simulink model "FreePortComm_RXTX"  (Simulink 7.4)
settings: Solver=FixedStepDiscrete  SolverMode=SingleTasking  StartTime=0.0  StopTime=inf  FixedStep=.02  RelTol=1e-3
settings Model: Creator=Admin  LastModifiedBy=fw  SimulationMode=external  ExtModeTrigDuration=500
settings ConfigSet: Description=rtmc9s12target_R2009b
settings DataIOCC: SignalLoggingName=sigsOut
settings OptimizationCC: BooleanDataType=off  InitFltsAndDblsToZero=on  OptimizeModelRefInitCode=on  LifeSpan=1
settings DebuggingCC: SaveWithParameterizedLinksMsg=none  SignalResolutionControl=TryResolveAllWithWarning  SolverPrmCheckMsg=none  MultiTaskDSMMsg=warning  MultiTaskCondExecSysMsg=none  StrictBusMsg=None
settings HardwareCC: ProdBitPerInt=16  ProdEndianess=BigEndian  ProdWordSize=16  ProdHWDeviceType=Motorola HC12
settings RTWCC: SystemTargetFile=mc9s12.tlc  GenerateMakefile=off  TemplateMakefile=mc9s12.tmf  ProcessScript=mc9s12_make_rtw_hook  IncludeERTFirstTime=on
settings CodeAppCC: IgnoreCustomStorageClasses=off
settings STFCustomTargetCC: TargetFcnLib=ansi_tfl_tmw.mat  ModelReferenceCompliant=off  IncludeMdlTerminateFcn=off  ERTCustomFileBanners=on  SupportNonInlinedSFcns=off  CPPClassGenCompliant=on  SystemTargetFile=mc9s12.tlc
settings ERTTargetCC: TargetFcnLib=ansi_tfl_tmw.mat  MultiwordLength=2048  ModelReferenceCompliant=off  ParMdlRefBuildCompliant=off  CompOptLevelCompliant=off  IncludeMdlTerminateFcn=off  CombineOutputUpdateFcns=off  ERTFirstTimeCompliant=off  SupportContinuousTime=on  ModelStepFunctionPrototypeControlCompliant=off  ExtModeMexFile=ext_serial_mc9s12_comm  ExtModeMexArgs=1,2,115200  InlinedParameterPlacement=NonHierarchical  ERTCustomFileTemplate=mc9s12_file_process.tlc  GRTInterface=on  ConvertIfToSwitch=off
settings CustomProperty: DataType=RTWOptions_EnumType_C__Users_fw__SVN_rtmc9s12-target_trunk_rtmc9s12_CW_R2009b_bin_mc9s12_1mc9s12_TargetBoard  Value=Dragon12Plus
settings EnumStrPairs: String=Dragon12

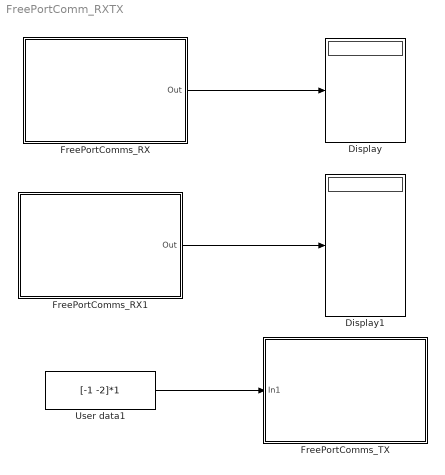
== system FreePortComm_RXTX ==
  Display : Display
  Display1 : Display
  FreePortComms_RX : Subsystem  Tag=mcTarget_freePortCommsRX  mask{sampletime=0.1, port=SCI0, baudrate=115200, channel=0, buf_size=5, data_type=UINT8, format=off, outformat=on}
      mask prompts: sampletime "Sample time"; port "Communication port"; channel "Channel number"; buf_size "Number of elements"; data_type "Data Type"; format "Block receives raw data"; outformat "Block output is double"
      mask init:
      | [buf_sizestr, portNamestr, baudratestr, channelstr, data_type_str, sampletime_str] = mbc_freeportrxd(sampletime, port, baudrate, channel, buf_size, data_type, format, outformat);
      mask Help: web('freePortComms_rxd.html');
      mask StyleString: edit,popup(SCI0|SCI1|COM1|COM2|COM3|COM4),popup(300|600|1200|2400|4800|9600|19200|38400|57600|115200),edit,edit,popup(SINGLE|INT8|UINT8|INT16|UINT16|INT32|UINT32|BOOLEAN),checkbox,checkbox
      mask Display: fprintf('Receive %s element(s)\nComm port: %s\nBaudrate: %s bps\nChannel: %s\nData type: %s\n Sample rate: %s', buf_sizestr, portNamestr, baudratestr, channelstr, data_type_str, sampletime_str)
  FreePortComms_RX1 : Subsystem  Tag=mcTarget_freePortCommsRX  mask{sampletime=0.1, port=SCI0, baudrate=115200, channel=1, buf_size=7, data_type=SINGLE, format=off, outformat=on}
      mask prompts: sampletime "Sample time"; port "Communication port"; channel "Channel number"; buf_size "Number of elements"; data_type "Data Type"; format "Block receives raw data"; outformat "Block output is double"
      mask init:
      | [buf_sizestr, portNamestr, baudratestr, channelstr, data_type_str, sampletime_str] = mbc_freeportrxd(sampletime, port, baudrate, channel, buf_size, data_type, format, outformat);
      mask Help: web('freePortComms_rxd.html');
      mask StyleString: edit,popup(SCI0|SCI1|COM1|COM2|COM3|COM4),popup(300|600|1200|2400|4800|9600|19200|38400|57600|115200),edit,edit,popup(SINGLE|INT8|UINT8|INT16|UINT16|INT32|UINT32|BOOLEAN),checkbox,checkbox
      mask Display: fprintf('Receive %s element(s)\nComm port: %s\nBaudrate: %s bps\nChannel: %s\nData type: %s\n Sample rate: %s', buf_sizestr, portNamestr, baudratestr, channelstr, data_type_str, sampletime_str)
  FreePortComms_TX : Subsystem  Tag=mcTarget_freePortCommsTX  mask{sampletime=0.1, port=SCI0, baudrate=115200, channel=3, buf_size=2, data_type=INT32, format=off}
      mask prompts: sampletime "Sample time"; port "Communication port"; channel "Channel number"; buf_size "Number of elements"; data_type "Data Type"; format "Block sends raw data"
      mask init:
      | [buf_sizestr, portNamestr, baudratestr, channelstr, data_type_str, sampletime_str] = mbc_freeporttxd(sampletime, port, baudrate, channel, buf_size, data_type, format);
      mask Help: web('freePortComms_txd.html');
      mask StyleString: edit,popup(SCI0|SCI1|COM1|COM2|COM3|COM4),popup(300|600|1200|2400|4800|9600|19200|38400|57600|115200),edit,edit,popup(SINGLE|INT8|UINT8|INT16|UINT16|INT32|UINT32|BOOLEAN),checkbox
      mask Display: fprintf('Transmit %s element(s)\nComm port: %s\nBaudrate: %s bps\nChannel: %s\nData type: %s\n Sample rate: %s', buf_sizestr, portNamestr, baudratestr, channelstr, data_type_str, sampletime_str)
  User data1 : Constant  Value=[-1 -2]*1  OutDataType=sfix(16)  OutScaling=2^0
  wires:
  FreePortComms_RX/1(Out) -> Display/1
  FreePortComms_RX1/1(Out) -> Display1/1
  User data1/1 -> FreePortComms_TX/1(In1)

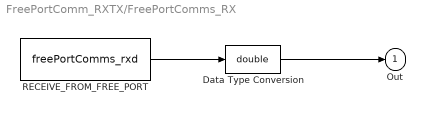
== system FreePortComm_RXTX/FreePortComms_RX ==
  Data Type Conversion : DataTypeConversion  OutDataTypeMode=double  OutDataType=sfix(16)  OutScaling=2^0  OutDataTypeStr=double  SaturateOnIntegerOverflow=on  RndMeth=Zero
  RECEIVE_FROM_FREE_PORT : S-Function  Tag=mcTarget_freePortCommsRX  FunctionName=freePortComms_rxd  Parameters=sampletime, channel, buf_size, data_type, port, baudrate, format  EnableBusSupport=off
  Out : Outport  OutDataType=sfix(16)  OutScaling=2^0
  wires:
  RECEIVE_FROM_FREE_PORT/1 -> Data Type Conversion/1
  Data Type Conversion/1 -> Out/1

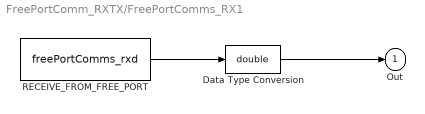
== system FreePortComm_RXTX/FreePortComms_RX1 ==
  Data Type Conversion : DataTypeConversion  OutDataTypeMode=double  OutDataType=sfix(16)  OutScaling=2^0  OutDataTypeStr=double  SaturateOnIntegerOverflow=on  RndMeth=Zero
  RECEIVE_FROM_FREE_PORT : S-Function  Tag=mcTarget_freePortCommsRX  FunctionName=freePortComms_rxd  Parameters=sampletime, channel, buf_size, data_type, port, baudrate, format  EnableBusSupport=off
  Out : Outport  OutDataType=sfix(16)  OutScaling=2^0
  wires:
  Data Type Conversion/1 -> Out/1
  RECEIVE_FROM_FREE_PORT/1 -> Data Type Conversion/1

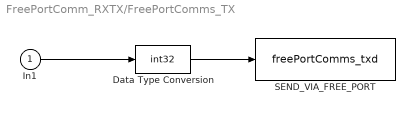
== system FreePortComm_RXTX/FreePortComms_TX ==
  In1 : Inport  OutDataType=sfix(16)  OutScaling=2^0
  Data Type Conversion : DataTypeConversion  OutDataTypeMode=int32  OutDataType=sfix(16)  OutScaling=2^0  OutDataTypeStr=int32  SaturateOnIntegerOverflow=on  RndMeth=Zero
  SEND_VIA_FREE_PORT : S-Function  Tag=mcTarget_freePortCommsTX  FunctionName=freePortComms_txd  Parameters=sampletime, channel, buf_size, data_type, port, baudrate, format  EnableBusSupport=off
  wires:
  In1/1 -> Data Type Conversion/1
  Data Type Conversion/1 -> SEND_VIA_FREE_PORT/1
